simulink model "my_PLL_IntegerN_transfer_model"  (R2024b)
settings: Solver=VariableStepAuto  StartTime=0.0  StopTime=10e-6  RelTol=1e-3
settings Model: Creator=BrunoFraga  LastModifiedBy=BrunoFraga

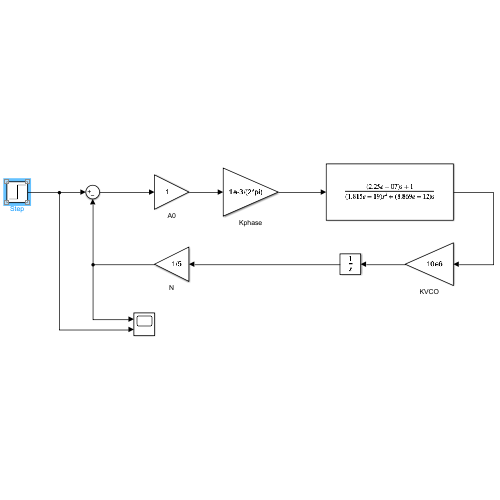
[thumbnail: Simulink's stored preview of the top-level diagram]
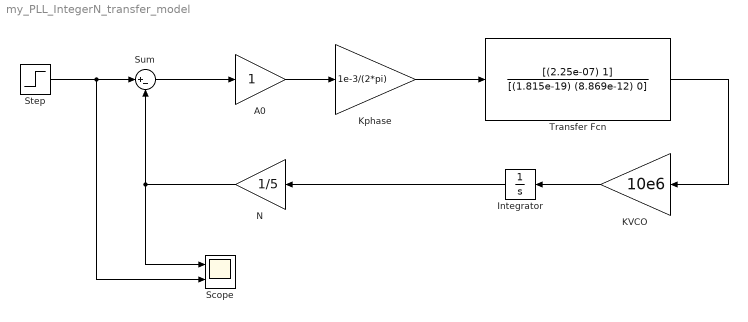
== system my_PLL_IntegerN_transfer_model ==
  A0 : Gain
  Integrator : Integrator
  KVCO : Gain  Gain=10e6
  Kphase : Gain  Gain=1e-3/(2*pi)
  N : Gain  Gain=1/5
  Scope : Scope  NumInputPorts=2
  Step : Step  Time=1e-6  SampleTime=0
  Sum : Sum  Inputs=|+-
  Transfer Fcn : TransferFcn  Numerator=[(2.25e-07) 1]  Denominator=[(1.815e-19) (8.869e-12) 0]
  wires:
  A0/1 -> Kphase/1
  Kphase/1 -> Transfer Fcn/1
  N/1 -> Sum/2, Scope/1
  Integrator/1 -> N/1
  KVCO/1 -> Integrator/1
  Sum/1 -> A0/1
  Transfer Fcn/1 -> KVCO/1
  Step/1 -> Scope/2, Sum/1
